simulink model "DSPB_MB_SS"  (Simulink 8.1)
settings: Solver=VariableStepDiscrete  StartTime=0.0  StopTime=DSPB_MB_SS_param.endTime  RelTol=1e-3
PreLoadFcn:
  | % Run the setup script when the model is opened
  | setup_DSPB_MB_SS;
InitFcn:
  | % Run the setup script again just before the
  | % model is run, so that any updates made
  | % after opening are applied.
  | setup_DSPB_MB_SS;
undefined symbols (not defined in the file or in its folder): a, AdvDSPBDMemDisplay, dpoly, DSPB_MB_SS_param, dspba, evalAionMaskParam, primtype, UseDontCare, value, x, y
libraries: DSPBAPrim x298, DspbAdvFftLibrary x34, DSPBABase x5, simulink x3, DSPBAModelBus x3, DSPBAVectorUtil x3, DSPBAControl x2
(part 2 of 4)

== system DSPB_MB_SS/dut/Output_Interface/addr_counter1 ==
  en : Inport
  CmpEQ : DSPBAPrim/CmpEQ  primtype=cmpeq  nInputs=2  nOutputs=1  omode=boolean  otype=sfix(16)  scale=2^-15  rndmethod=Unbiased  factor=1  satmethod=Symmetric  shift_vec=[0 1 2 -1]  value=0  inPortNames=[' '; ' ';]  outPortNames=[' ']  dspbaimage=dspba_prim.jpg  text=fprintf('==');  style=Optimised  visibilities=0  advOptions=[]  version=20130117
  Const1 : DSPBAPrim/Const  primtype=const  nInputs=0  nOutputs=1  omode=Specify via dialog  otype=ufix(DSPB_MB_SS_param.FS+1)  scale=2^-0  rndmethod=Unbiased  factor=1  satmethod=Symmetric  shift_vec=[0 1 2 -1]  value=2^(DSPB_MB_SS_param.FS) + 1  inPortNames=['+'; '+';]  outPortNames=[' ']  dspbaimage=dspba_prim.jpg  text=fprintf('%s', num2str(value));  style=Optimised  visibilities=8 + 1024  floatPrecision=float32_m23  version=20120820
  Const2 : DSPBAPrim/Const  primtype=const  nInputs=0  nOutputs=1  omode=Specify via dialog  otype=ufix(DSPB_MB_SS_param.FS + 1)  scale=2^-0  rndmethod=Unbiased  factor=1  satmethod=Symmetric  shift_vec=[0 1 2 -1]  value=2^(DSPB_MB_SS_param.FS)  inPortNames=['+'; '+';]  outPortNames=[' ']  dspbaimage=dspba_prim.jpg  text=fprintf('%s', num2str(value));  style=Optimised  visibilities=8 + 1024  floatPrecision=float32_m23  version=20120820
  Const3 : DSPBAPrim/Const  primtype=const  nInputs=0  nOutputs=1  omode=boolean  otype=ufix(10)  scale=2^-0  rndmethod=Unbiased  factor=1  satmethod=Symmetric  shift_vec=[0 1 2 -1]  value=1  inPortNames=['+'; '+';]  outPortNames=[' ']  dspbaimage=dspba_prim.jpg  text=fprintf('%s', num2str(value));  style=Optimised  visibilities=8 + 1024  floatPrecision=float32_m23  version=20120820
  Const4 : DSPBAPrim/Const  primtype=const  nInputs=0  nOutputs=1  omode=Inherit via internal rule  otype=ufix(10)  scale=2^-0  rndmethod=Unbiased  factor=1  satmethod=Symmetric  shift_vec=[0 1 2 -1]  value=0  inPortNames=['+'; '+';]  outPortNames=[' ']  dspbaimage=dspba_prim.jpg  text=fprintf('%s', num2str(value));  style=Optimised  visibilities=8 + 1024  floatPrecision=float32_m23  version=20120820
  LoadableCounter : DSPBAPrim/LoadableCounter  primtype=loadablecounter  nInputs=5  nOutputs=1  omode=Specify via dialog  otype=ufix(DSPB_MB_SS_param.FS+1)  scale=2^-0  rndmethod=Unbiased  factor=1  satmethod=Symmetric  shift_vec=[0 1 2 -1]  value=[0 2^(DSPB_MB_SS_param.FS) + 1 1]  inPortNames=['en';'ld';'i ';'s ';'m ']  outPortNames=[' ']  dspbaimage=dspba_prim.jpg  text=fprintf('loadable\ncounter\n[%d %d %d]', value(1), value(2), value(3));  style=Optimised  visibilities=8 + 1024  version=20090407
  SampleDelay : DSPBAPrim/SampleDelay  primtype=sampdelay  nInputs=1  nOutputs=1  omode=Inherit via internal rule  otype=sfix(16)  scale=2^-15  rndmethod=Unbiased  factor=1  satmethod=Symmetric  shift_vec=[0 1 2 -1]  value=1  inPortNames=[' '; ' ';]  outPortNames=[' ']  dspbaimage=dspba_prim.jpg  text=dpoly(1, eye(1,value+1), 'z')  style=Optimised  visibilities=8 + 1024 + 2^17 + 2^18  flexible=off  slackgroup=0  augmented=0  version=20090407  advOptions=[]
  count : Outport
  wires:
  Const2/1 -> CmpEQ/2
  CmpEQ/1 -> SampleDelay/1
  Const4/1 -> LoadableCounter/3
  Const1/1 -> LoadableCounter/5
  SampleDelay/1 -> LoadableCounter/2
  Const3/1 -> LoadableCounter/4
  en/1 -> LoadableCounter/1
  LoadableCounter/1 -> count/1, CmpEQ/1

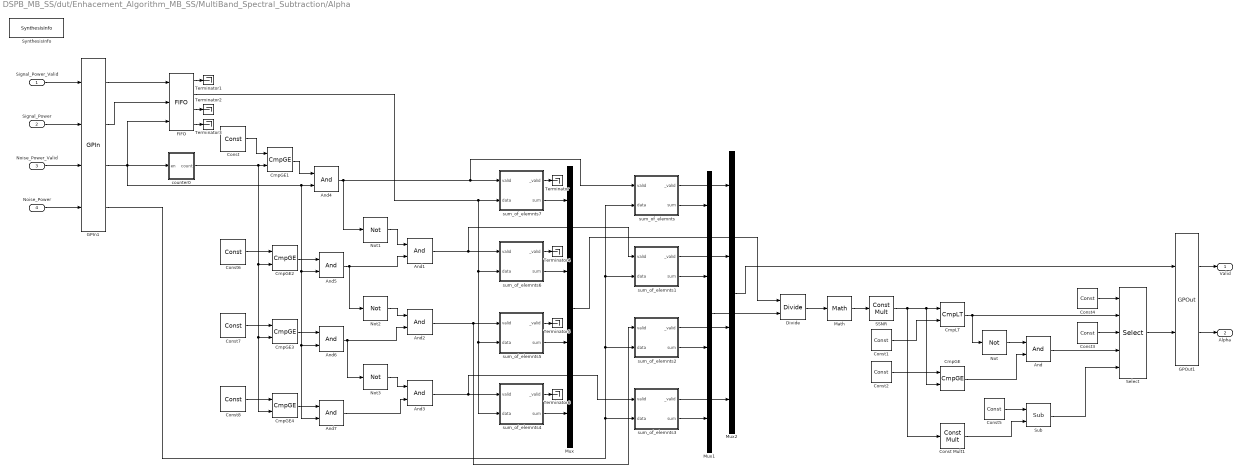
== system DSPB_MB_SS/dut/Enhacement_Algorithm_MB_SS/MultiBand_Spectral_Subtraction/Alpha ==
  Signal_Power_Valid : Inport
  Signal_Power : Inport  Port=2
  Noise_Power_Valid : Inport  Port=3
  Noise_Power : Inport  Port=4
  And{,1..7} (8 alike) : DSPBAPrim/And  primtype=and  nInputs=2  nOutputs=1  omode=Inherit via internal rule  otype=sfix(16)  scale=2^-15  rndmethod=Unbiased  factor=1  satmethod=Symmetric  shift_vec=[0 1 2 -1]  value=0  inPortNames=[' '; ' '; ' '; ' '; ' '; ' '; ' '; ' '; ' '; ' '; ' '; ' '; ' '; ' '; ' '; ' '; ]  outPortNames=[' ']  dspbaimage=dspba_prim.jpg  text=fprintf('&');  style=Optimised  visibilities=8+2  version=20090407
  CmpGE{,1..4} (5 alike) : DSPBAPrim/CmpGE  primtype=cmpgte  nInputs=2  nOutputs=1  omode=boolean  otype=sfix(16)  scale=2^-15  rndmethod=Unbiased  factor=1  satmethod=Symmetric  shift_vec=[0 1 2 -1]  value=0  inPortNames=['a'; 'b';]  outPortNames=[' ']  dspbaimage=dspba_prim.jpg  text=fprintf('a>=b');  style=Optimised  visibilities=0  advOptions=[]  version=20130117
  CmpLT : DSPBAPrim/CmpLT  primtype=cmplt  nInputs=2  nOutputs=1  omode=boolean  otype=sfix(16)  scale=2^-15  rndmethod=Unbiased  factor=1  satmethod=Symmetric  shift_vec=[0 1 2 -1]  value=0  inPortNames=['a'; 'b';]  outPortNames=[' ']  dspbaimage=dspba_prim.jpg  text=fprintf('a<b');  style=Optimised  visibilities=0  advOptions=[]  version=20130117
  Const : DSPBAPrim/Const  primtype=const  nInputs=0  nOutputs=1  omode=Specify via dialog  otype=ufix(10)  scale=2^-0  rndmethod=Unbiased  factor=1  satmethod=Symmetric  shift_vec=[0 1 2 -1]  value=2^(DSPB_MB_SS_param.FS-1-log2(DSPB_MB_SS_param.NB))  inPortNames=['+'; '+';]  outPortNames=[' ']  dspbaimage=dspba_prim.jpg  text=fprintf('%s', num2str(value));  style=Optimised  visibilities=8 + 1024  floatPrecision=float32_m23  version=20120820
  Const Mult1 : DSPBAPrim/Const Mult  primtype=constmult  nInputs=1  nOutputs=1  omode=Inherit via internal rule  otype=sfix(16)  scale=2^-15  rndmethod=Unbiased  factor=1  satmethod=Symmetric  shift_vec=[0 1 2 -1]  value=3/20  inPortNames=[' '; ' ';]  outPortNames=[' ']  dspbaimage=dspba_prim.jpg  text=fprintf('cx');  style=Optimised  visibilities=8+2^10+2^17+2^18  floatRounding=correct  advOptions=[]  version=20140218
  Const1 : DSPBAPrim/Const  primtype=const  nInputs=0  nOutputs=1  omode=single  otype=sfix(16)  scale=2^-15  rndmethod=Unbiased  factor=1  satmethod=Symmetric  shift_vec=[0 1 2 -1]  value=-5  inPortNames=['+'; '+';]  outPortNames=[' ']  dspbaimage=dspba_prim.jpg  text=fprintf('%s', num2str(value));  style=Optimised  visibilities=8 + 1024  floatPrecision=float32_m23  version=20120820
  Const2 : DSPBAPrim/Const  primtype=const  nInputs=0  nOutputs=1  omode=single  otype=sfix(16)  scale=2^-15  rndmethod=Unbiased  factor=1  satmethod=Symmetric  shift_vec=[0 1 2 -1]  value=20  inPortNames=['+'; '+';]  outPortNames=[' ']  dspbaimage=dspba_prim.jpg  text=fprintf('%s', num2str(value));  style=Optimised  visibilities=8 + 1024  floatPrecision=float32_m23  version=20120820
  Const3 : DSPBAPrim/Const  primtype=const  nInputs=0  nOutputs=1  omode=single  otype=sfix(16)  scale=2^-15  rndmethod=Unbiased  factor=1  satmethod=Symmetric  shift_vec=[0 1 2 -1]  value=5  inPortNames=['+'; '+';]  outPortNames=[' ']  dspbaimage=dspba_prim.jpg  text=fprintf('%s', num2str(value));  style=Optimised  visibilities=8 + 1024  floatPrecision=float32_m23  version=20120820
  Const4 : DSPBAPrim/Const  primtype=const  nInputs=0  nOutputs=1  omode=single  otype=sfix(16)  scale=2^-15  rndmethod=Unbiased  factor=1  satmethod=Symmetric  shift_vec=[0 1 2 -1]  value=1  inPortNames=['+'; '+';]  outPortNames=[' ']  dspbaimage=dspba_prim.jpg  text=fprintf('%s', num2str(value));  style=Optimised  visibilities=8 + 1024  floatPrecision=float32_m23  version=20120820
  Const5 : DSPBAPrim/Const  primtype=const  nInputs=0  nOutputs=1  omode=single  otype=sfix(16)  scale=2^-15  rndmethod=Unbiased  factor=1  satmethod=Symmetric  shift_vec=[0 1 2 -1]  value=4  inPortNames=['+'; '+';]  outPortNames=[' ']  dspbaimage=dspba_prim.jpg  text=fprintf('%s', num2str(value));  style=Optimised  visibilities=8 + 1024  floatPrecision=float32_m23  version=20120820
  Const6 : DSPBAPrim/Const  primtype=const  nInputs=0  nOutputs=1  omode=Specify via dialog  otype=ufix(10)  scale=2^-0  rndmethod=Unbiased  factor=1  satmethod=Symmetric  shift_vec=[0 1 2 -1]  value=2*2^(DSPB_MB_SS_param.FS-1-log2(DSPB_MB_SS_param.NB))  inPortNames=['+'; '+';]  outPortNames=[' ']  dspbaimage=dspba_prim.jpg  text=fprintf('%s', num2str(value));  style=Optimised  visibilities=8 + 1024  floatPrecision=float32_m23  version=20120820
  Const7 : DSPBAPrim/Const  primtype=const  nInputs=0  nOutputs=1  omode=Specify via dialog  otype=ufix(10)  scale=2^-0  rndmethod=Unbiased  factor=1  satmethod=Symmetric  shift_vec=[0 1 2 -1]  value=3*2^(DSPB_MB_SS_param.FS-1-log2(DSPB_MB_SS_param.NB))  inPortNames=['+'; '+';]  outPortNames=[' ']  dspbaimage=dspba_prim.jpg  text=fprintf('%s', num2str(value));  style=Optimised  visibilities=8 + 1024  floatPrecision=float32_m23  version=20120820
  Const8 : DSPBAPrim/Const  primtype=const  nInputs=0  nOutputs=1  omode=Specify via dialog  otype=ufix(10)  scale=2^-0  rndmethod=Unbiased  factor=1  satmethod=Symmetric  shift_vec=[0 1 2 -1]  value=4*2^(DSPB_MB_SS_param.FS-1-log2(DSPB_MB_SS_param.NB))  inPortNames=['+'; '+';]  outPortNames=[' ']  dspbaimage=dspba_prim.jpg  text=fprintf('%s', num2str(value));  style=Optimised  visibilities=8 + 1024  floatPrecision=float32_m23  version=20120820
  Divide : DSPBAPrim/Divide  primtype=divide  nInputs=2  nOutputs=1  omode=Inherit via internal rule  otype=sfix(16)  scale=2^-15  rndmethod=Unbiased  factor=1  satmethod=Symmetric  shift_vec=[0 1 2 -1]  value=round([0:255]/17)  inPortNames=[' '; ' ';]  outPortNames=[' ']  dspbaimage=dspba_prim.jpg  text=fprintf('a\n----\nb');  style=Optimised  visibilities=8+2^17+2^18  floatRounding=correct  advOptions=[]  version=20130115
  FIFO : DSPBAPrim/FIFO  primtype=fifo  nInputs=3  nOutputs=4  omode=Inherit via internal rule  otype=sfix(16)  scale=2^-15  rndmethod=Unbiased  factor=1  satmethod=Symmetric  shift_vec=[0 1 2 -1]  value=[2^(DSPB_MB_SS_param.FS-1) 1 2^(DSPB_MB_SS_param.FS-1)]  inPortNames=['w'; 'd'; 'r'; 'f']  outPortNames=['v'; 'q'; 't'; 'f']  dspbaimage=dspba_prim.jpg  text=fprintf('fifo');  style=Optimised  visibilities=263168  version=20130808  user_sclr=off
  GPIn1 : DSPBAPrim/GPIn  primtype=gpin  nInputs=evalAionMaskParam(gcb,'value',1)  nOutputs=evalAionMaskParam(gcb,'value',1)  omode=Inherit via internal rule  otype=sfix(16)  scale=2^-15  rndmethod=Unbiased  factor=1  satmethod=Symmetric  shift_vec=[0 1 2 -1]  value=4  inPortNames=[' ' ' ' ' ' ' ' ' ' ' ' ' ' ' ' ' ' ' ' ' ' ' ' ' ' ' ' ' ' ' ' ' ' ' ' ' ' ' ' ' ' ' ' ' ' ' ' ' ' ' ' ' ' ' ' ' ' ' ' ' ' ' ' ' ' ' ' ' ']'  outPortNames=[' ' ' ' ' ' ' ' ' ' ' ' ' ' ' ' ' ' ' ' ' ' ' ' ' ' ' ' ' ' ' ' ' ' ' ' ' ' ' ' ' ' ' ' ' ' ' ' ' ' ' ' ' ' ' ' ' ' ' ' ' ' ' ' ' ' ' ' ' ']'  dspbaimage=dspba_prim.jpg  text=fprintf('GPIn');  style=Optimised  visibilities=1024  latencyCorrection=0  scheduleOrigin=on  version=20090407
  GPOut1 : DSPBAPrim/GPOut  primtype=gpout  nInputs=evalAionMaskParam(gcb,'value',1)  nOutputs=evalAionMaskParam(gcb,'value',1)  omode=Inherit via internal rule  otype=sfix(16)  scale=2^-15  rndmethod=Unbiased  factor=1  satmethod=Symmetric  shift_vec=[0 1 2 -1]  value=2  inPortNames=[' ' ' ' ' ' ' ' ' ' ' ' ' ' ' ' ' ' ' ' ' ' ' ' ' ' ' ' ' ' ' ' ' ' ' ' ' ' ' ' ' ' ' ' ' ' ' ' ' ' ' ' ' ' ' ' ' ' ' ' ' ' ' ' ' ' ' ' ' ']'  outPortNames=[' ' ' ' ' ' ' ' ' ' ' ' ' ' ' ' ' ' ' ' ' ' ' ' ' ' ' ' ' ' ' ' ' ' ' ' ' ' ' ' ' ' ' ' ' ' ' ' ' ' ' ' ' ' ' ' ' ' ' ' ' ' ' ' ' ' ' ' ' ']'  dspbaimage=dspba_prim.jpg  text=fprintf('GPOut');  style=Optimised  visibilities=1024  latencyCorrection=0  version=20090407
  Math : DSPBAPrim/Math  primtype=mathfunc  nInputs=1  nOutputs=1  omode=Inherit via internal rule  otype=sfix(16)  scale=2^-15  rndmethod=Unbiased  factor=1  satmethod=Symmetric  shift_vec=[0 1 2 -1]  value=round([0:255]/17)  inPortNames=[' '; ' ';]  outPortNames=[' ']  dspbaimage=dspba_prim_float.jpg  text=fprintf('exp(x)');  style=Optimised  visibilities=2^17  functionExpr=log10(x)  advOptions=[]  floatRounding=correct  version=20130910
  Mux : Mux
  Mux1 : Mux
  Mux2 : Mux
  Not{,1..3} (4 alike) : DSPBAPrim/Not  primtype=not  nInputs=1  nOutputs=1  omode=Inherit via internal rule  otype=sfix(16)  scale=2^-15  rndmethod=Unbiased  factor=1  satmethod=Symmetric  shift_vec=[0 1 2 -1]  value=0  inPortNames=[' '; ' ';]  outPortNames=[' ']  dspbaimage=dspba_prim.jpg  text=fprintf('~');  style=Optimised  visibilities=8  version=20090407
  SSNR : DSPBAPrim/Const Mult  primtype=constmult  nInputs=1  nOutputs=1  omode=Inherit via internal rule  otype=sfix(16)  scale=2^-15  rndmethod=Unbiased  factor=1  satmethod=Symmetric  shift_vec=[0 1 2 -1]  value=10  inPortNames=[' '; ' ';]  outPortNames=[' ']  dspbaimage=dspba_prim.jpg  text=fprintf('cx');  style=Optimised  visibilities=8+2^10+2^17+2^18  floatRounding=correct  advOptions=[]  version=20140218
  Select : DSPBAPrim/Select  primtype=select  nInputs=str2num(get_param(gcb,'value'))*2+1  nOutputs=1  omode=Inherit via internal rule  otype=sfix(16)  scale=2^-15  rndmethod=Unbiased  factor=1  satmethod=Symmetric  shift_vec=[0 1 2 -1]  value=2  inPortNames=['d'; '0'; 'a'; '1'; 'b'; '2'; 'c'; '3'; 'd'; '4'; 'e'; '5'; 'f'; '6'; 'g'; '7'; 'h'; '8'; 'i'; '9'; 'j']  outPortNames=[' ']  dspbaimage=dspba_prim.jpg  text=fprintf('%s', primtype);  style=Optimised  visibilities=8 + 1024  version=20090407
  Sub : DSPBAPrim/Sub  primtype=sub  nInputs=2  nOutputs=1  omode=Inherit via internal rule with word growth  otype=sfix(16)  scale=2^-15  rndmethod=Unbiased  factor=1  satmethod=Symmetric  shift_vec=[0 1 2 -1]  value=0  inPortNames=['+'; '-';]  outPortNames=[' ']  dspbaimage=dspba_prim.jpg  text=fprintf('-');  style=Optimised  visibilities=8+2^17+2^18  floatRounding=correct  advOptions=[]  version=20130115
  SynthesisInfo : DSPBAPrim/SynthesisInfo  primtype=synthinfo  nInputs=0  nOutputs=0  omode=Inherit via internal rule  otype=sfix(16)  scale=2^-15  rndmethod=Truncate  factor=1  satmethod=Symmetric  shift_vec=[0 1 2 -1]  value=99  inPortNames=[' '; ' ';]  outPortNames=[' ']  dspbaimage=dspba_prim_ctrl.jpg  text=fprintf('Style=%s', style);  style=Scheduled  visibilities=2^17+2^18+2^19+2^20  constraintInUse=off  constraintRelation==  constraintLimit=5  bitAccurate=on  version=20150220
  Terminator{,1..6} (7 alike) : Terminator
  counter0 : Subsystem
  sum_of_elemnts : Subsystem
  sum_of_elemnts1 : Subsystem
  sum_of_elemnts2 : Subsystem
  sum_of_elemnts3 : Subsystem
  sum_of_elemnts4 : Subsystem
  sum_of_elemnts5 : Subsystem
  sum_of_elemnts6 : Subsystem
  sum_of_elemnts7 : Subsystem
  Valid : Outport
  Alpha : Outport  Port=2
  wires:
  Math/1 -> SSNR/1
  SSNR/1 -> Const Mult1/1, CmpGE/2, CmpLT/1
  Const1/1 -> CmpLT/2
  CmpLT/1 -> Not/1, Select/2
  Const2/1 -> CmpGE/1
  Not/1 -> And/1
  CmpGE/1 -> And/2
  And/1 -> Select/4
  Const3/1 -> Select/3
  Const4/1 -> Select/1
  Const5/1 -> Sub/1
  Const Mult1/1 -> Sub/2
  Sub/1 -> Select/5
  Signal_Power_Valid/1 -> GPIn1/1
  Signal_Power/1 -> GPIn1/2
  Noise_Power/1 -> GPIn1/4
  Noise_Power_Valid/1 -> GPIn1/3
  GPIn1/2 -> FIFO/2
  GPIn1/1 -> FIFO/1
  Const/1 -> CmpGE1/1
  counter0/1(count) -> CmpGE1/2, CmpGE2/2, CmpGE4/2, CmpGE3/2
  GPIn1/3 -> And7/2, And6/2, And5/2, And4/2, counter0/1(en), FIFO/3
  Not1/1 -> And1/1
  Not2/1 -> And2/1
  Const6/1 -> CmpGE2/1
  Const7/1 -> CmpGE3/1
  And5/1 -> And1/2, Not2/1
  Not3/1 -> And3/1
  CmpGE2/1 -> And5/1
  And6/1 -> Not3/1, And2/2
  And7/1 -> And3/2
  CmpGE3/1 -> And6/1
  CmpGE4/1 -> And7/1
  Const8/1 -> CmpGE4/1
  CmpGE1/1 -> And4/1
  And4/1 -> Not1/1, sum_of_elemnts7/1(valid), sum_of_elemnts/1(valid)
  And1/1 -> sum_of_elemnts6/1(valid), sum_of_elemnts1/1(valid)
  And2/1 -> sum_of_elemnts5/1(valid), sum_of_elemnts2/1(valid)
  And3/1 -> sum_of_elemnts4/1(valid), sum_of_elemnts3/1(valid)
  FIFO/2 -> sum_of_elemnts7/2(data), sum_of_elemnts6/2(data), sum_of_elemnts5/2(data), sum_of_elemnts4/2(data)
  GPIn1/4 -> sum_of_elemnts3/2(data), sum_of_elemnts2/2(data), sum_of_elemnts1/2(data), sum_of_elemnts/2(data)
  Divide/1 -> Math/1
  FIFO/1 -> Terminator1/1
  FIFO/3 -> Terminator2/1
  FIFO/4 -> Terminator3/1
  sum_of_elemnts7/2(sum) -> Mux/1
  sum_of_elemnts6/2(sum) -> Mux/2
  sum_of_elemnts4/2(sum) -> Mux/4
  sum_of_elemnts5/2(sum) -> Mux/3
  sum_of_elemnts/2(sum) -> Mux1/1
  sum_of_elemnts3/2(sum) -> Mux1/4
  sum_of_elemnts2/2(sum) -> Mux1/3
  sum_of_elemnts1/2(sum) -> Mux1/2
  Mux/1 -> Divide/1
  Mux1/1 -> Divide/2
  sum_of_elemnts7/1(_valid) -> Terminator/1
  sum_of_elemnts6/1(_valid) -> Terminator4/1
  sum_of_elemnts5/1(_valid) -> Terminator5/1
  sum_of_elemnts4/1(_valid) -> Terminator6/1
  GPOut1/1 -> Valid/1
  GPOut1/2 -> Alpha/1
  Select/1 -> GPOut1/2
  sum_of_elemnts/1(_valid) -> Mux2/1
  sum_of_elemnts1/1(_valid) -> Mux2/2
  sum_of_elemnts2/1(_valid) -> Mux2/3
  sum_of_elemnts3/1(_valid) -> Mux2/4
  Mux2/1 -> GPOut1/1

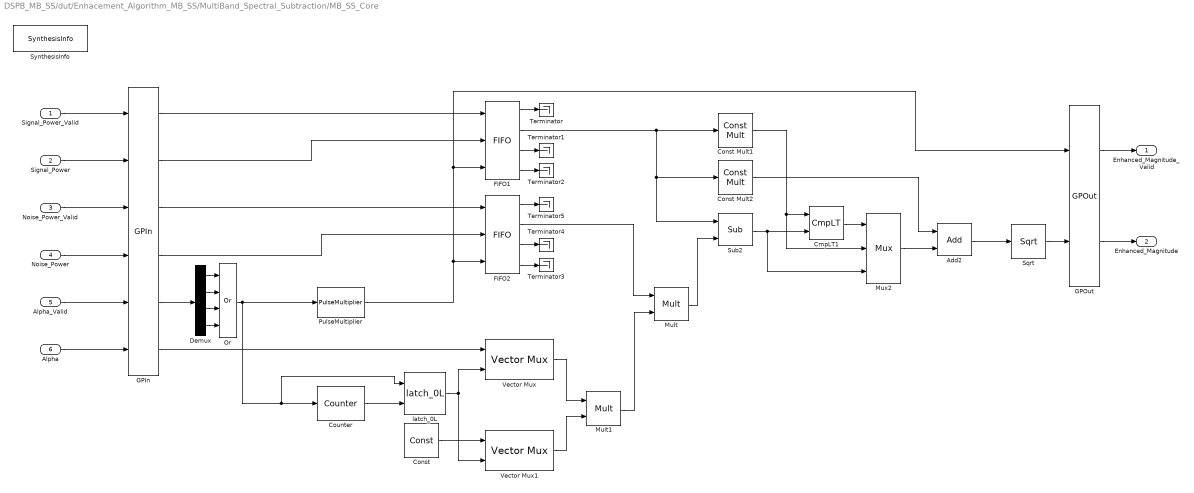
== system DSPB_MB_SS/dut/Enhacement_Algorithm_MB_SS/MultiBand_Spectral_Subtraction/MB_SS_Core ==
  Signal_Power_Valid : Inport
  Signal_Power : Inport  Port=2
  Noise_Power_Valid : Inport  Port=3
  Noise_Power : Inport  Port=4
  Alpha_Valid : Inport  Port=5
  Alpha : Inport  Port=6
  Add2 : DSPBAPrim/Add  primtype=add  nInputs=evalAionMaskParam(gcb,'value',1)  nOutputs=1  omode=Inherit via internal rule  otype=ufix(DSPB_MB_SS_param.FS + 1)  scale=2^-0  rndmethod=Unbiased  factor=1  satmethod=Symmetric  shift_vec=[0 1 2 -1]  value=2  inPortNames=[' '; ' ';]  outPortNames=[' ']  dspbaimage=dspba_prim.jpg  text=fprintf('+');  style=Optimised  visibilities=1032+2^17+2^18+2^19  genFPC=off  floatRounding=correct  advOptions=[]  version=20130821
  CmpLT1 : DSPBAPrim/CmpLT  primtype=cmplt  nInputs=2  nOutputs=1  omode=boolean  otype=sfix(16)  scale=2^-15  rndmethod=Unbiased  factor=1  satmethod=Symmetric  shift_vec=[0 1 2 -1]  value=0  inPortNames=['a'; 'b';]  outPortNames=[' ']  dspbaimage=dspba_prim.jpg  text=fprintf('a<b');  style=Optimised  visibilities=0  advOptions=[]  version=20130117
  Const : DSPBAPrim/Const  primtype=const  nInputs=0  nOutputs=1  omode=single  otype=sfix(16)  scale=2^-15  rndmethod=Unbiased  factor=1  satmethod=Symmetric  shift_vec=[0 1 2 -1]  value=[1 2.5 2.5 1.5]  inPortNames=['+'; '+';]  outPortNames=[' ']  dspbaimage=dspba_prim.jpg  text=fprintf('%s', num2str(value));  style=Optimised  visibilities=8 + 1024  floatPrecision=float32_m23  version=20120820
  Const Mult1 : DSPBAPrim/Const Mult  primtype=constmult  nInputs=1  nOutputs=1  omode=Inherit via internal rule  otype=sfix(16)  scale=2^-15  rndmethod=Unbiased  factor=1  satmethod=Symmetric  shift_vec=[0 1 2 -1]  value=0.002  inPortNames=[' '; ' ';]  outPortNames=[' ']  dspbaimage=dspba_prim.jpg  text=fprintf('cx');  style=Optimised  visibilities=8+2^10+2^17+2^18  floatRounding=correct  advOptions=[]  version=20140218
  Const Mult2 : DSPBAPrim/Const Mult  primtype=constmult  nInputs=1  nOutputs=1  omode=Inherit via internal rule  otype=sfix(16)  scale=2^-15  rndmethod=Unbiased  factor=1  satmethod=Symmetric  shift_vec=[0 1 2 -1]  value=0.05  inPortNames=[' '; ' ';]  outPortNames=[' ']  dspbaimage=dspba_prim.jpg  text=fprintf('cx');  style=Optimised  visibilities=8+2^10+2^17+2^18  floatRounding=correct  advOptions=[]  version=20140218
  Counter : DSPBAPrim/Counter  primtype=counter  nInputs=1  nOutputs=1  omode=Inherit via internal rule  otype=ufix(16)  scale=2^-0  rndmethod=Unbiased  factor=1  satmethod=Symmetric  shift_vec=[0 1 2 -1]  value=[DSPB_MB_SS_param.NB-1 DSPB_MB_SS_param.NB 1]  inPortNames=[' '; ' ';]  outPortNames=[' ']  dspbaimage=dspba_prim.jpg  text=fprintf('counter\n[%d %d %d]', value(1), value(2), value(3));  style=Optimised  visibilities=8 + 1024  version=20090407
  Demux : Demux
  FIFO1 : DSPBAPrim/FIFO  primtype=fifo  nInputs=3  nOutputs=4  omode=Inherit via internal rule  otype=sfix(16)  scale=2^-15  rndmethod=Unbiased  factor=1  satmethod=Symmetric  shift_vec=[0 1 2 -1]  value=[2^(DSPB_MB_SS_param.FS-1) 1 2^(DSPB_MB_SS_param.FS-1)]  inPortNames=['w'; 'd'; 'r'; 'f']  outPortNames=['v'; 'q'; 't'; 'f']  dspbaimage=dspba_prim.jpg  text=fprintf('fifo');  style=Optimised  visibilities=263168  version=20130808  user_sclr=off
  FIFO2 : DSPBAPrim/FIFO  primtype=fifo  nInputs=3  nOutputs=4  omode=Inherit via internal rule  otype=sfix(16)  scale=2^-15  rndmethod=Unbiased  factor=1  satmethod=Symmetric  shift_vec=[0 1 2 -1]  value=[2^(DSPB_MB_SS_param.FS-1) 1 2^(DSPB_MB_SS_param.FS-1)]  inPortNames=['w'; 'd'; 'r'; 'f']  outPortNames=['v'; 'q'; 't'; 'f']  dspbaimage=dspba_prim.jpg  text=fprintf('fifo');  style=Optimised  visibilities=263168  version=20130808  user_sclr=off
  GPIn : DSPBAPrim/GPIn  primtype=gpin  nInputs=evalAionMaskParam(gcb,'value',1)  nOutputs=evalAionMaskParam(gcb,'value',1)  omode=Inherit via internal rule  otype=sfix(16)  scale=2^-15  rndmethod=Unbiased  factor=1  satmethod=Symmetric  shift_vec=[0 1 2 -1]  value=6  inPortNames=[' ' ' ' ' ' ' ' ' ' ' ' ' ' ' ' ' ' ' ' ' ' ' ' ' ' ' ' ' ' ' ' ' ' ' ' ' ' ' ' ' ' ' ' ' ' ' ' ' ' ' ' ' ' ' ' ' ' ' ' ' ' ' ' ' ' ' ' ' ']'  outPortNames=[' ' ' ' ' ' ' ' ' ' ' ' ' ' ' ' ' ' ' ' ' ' ' ' ' ' ' ' ' ' ' ' ' ' ' ' ' ' ' ' ' ' ' ' ' ' ' ' ' ' ' ' ' ' ' ' ' ' ' ' ' ' ' ' ' ' ' ' ' ']'  dspbaimage=dspba_prim.jpg  text=fprintf('GPIn');  style=Optimised  visibilities=1024  latencyCorrection=0  scheduleOrigin=on  version=20090407
  GPOut : DSPBAPrim/GPOut  primtype=gpout  nInputs=evalAionMaskParam(gcb,'value',1)  nOutputs=evalAionMaskParam(gcb,'value',1)  omode=Inherit via internal rule  otype=sfix(16)  scale=2^-15  rndmethod=Unbiased  factor=1  satmethod=Symmetric  shift_vec=[0 1 2 -1]  value=2  inPortNames=[' ' ' ' ' ' ' ' ' ' ' ' ' ' ' ' ' ' ' ' ' ' ' ' ' ' ' ' ' ' ' ' ' ' ' ' ' ' ' ' ' ' ' ' ' ' ' ' ' ' ' ' ' ' ' ' ' ' ' ' ' ' ' ' ' ' ' ' ' ']'  outPortNames=[' ' ' ' ' ' ' ' ' ' ' ' ' ' ' ' ' ' ' ' ' ' ' ' ' ' ' ' ' ' ' ' ' ' ' ' ' ' ' ' ' ' ' ' ' ' ' ' ' ' ' ' ' ' ' ' ' ' ' ' ' ' ' ' ' ' ' ' ' ']'  dspbaimage=dspba_prim.jpg  text=fprintf('GPOut');  style=Optimised  visibilities=1024  latencyCorrection=0  version=20090407
  Mult : DSPBAPrim/Mult  primtype=mult  nInputs=2  nOutputs=1  omode=Inherit via internal rule  otype=sfix(16)  scale=2^-15  rndmethod=Unbiased  factor=1  satmethod=Symmetric  shift_vec=[0 1 2 -1]  value=0  inPortNames=[' '; ' ';]  outPortNames=[' ']  dspbaimage=dspba_prim.jpg  text=fprintf('X');  style=Optimised  visibilities=8+2^18+2^19  floatPrecision=float32_m23  floatRounding=correct  advOptions=[]  version=20130115
  Mult1 : DSPBAPrim/Mult  primtype=mult  nInputs=2  nOutputs=1  omode=Inherit via internal rule  otype=sfix(16)  scale=2^-15  rndmethod=Unbiased  factor=1  satmethod=Symmetric  shift_vec=[0 1 2 -1]  value=0  inPortNames=[' '; ' ';]  outPortNames=[' ']  dspbaimage=dspba_prim.jpg  text=fprintf('X');  style=Optimised  visibilities=8+2^18+2^19  floatPrecision=float32_m23  floatRounding=correct  advOptions=[]  version=20130115
  Mux2 : DSPBAPrim/Mux  primtype=mux  nInputs=evalAionMaskParam(gcb,'value',1)+1  nOutputs=1  omode=Inherit via internal rule  otype=sfix(16)  scale=2^-15  rndmethod=Unbiased  factor=1  satmethod=Symmetric  shift_vec=[0 1 2 -1]  value=2  inPortNames=['s '; 'd0'; 'd1'; 'd2'; 'd3'; 'd4'; 'd5'; 'd6'; 'd7'; 'd8'; 'd9';]  outPortNames=[' ']  dspbaimage=dspba_prim.jpg  text=fprintf('%s', primtype);  style=Optimised  visibilities=1032  version=20131025
  Or : DSPBAPrim/Or  primtype=or  nInputs=4  nOutputs=1  omode=Inherit via internal rule  otype=sfix(16)  scale=2^-15  rndmethod=Unbiased  factor=1  satmethod=Symmetric  shift_vec=[0 1 2 -1]  value=0  inPortNames=[' '; ' '; ' '; ' '; ' '; ' '; ' '; ' '; ' '; ' '; ' '; ' '; ' '; ' '; ' '; ' '; ]  outPortNames=[' ']  dspbaimage=dspba_prim.jpg  text=fprintf('|');  style=Optimised  visibilities=8+2  version=20090407
  PulseMultiplier : DspbAdvFftLibrary/Common/PulseMultiplier  N=DSPB_MB_SS_param.FS-1-log2(DSPB_MB_SS_param.NB)
  Sqrt : DSPBAPrim/Sqrt  primtype=sqrtfunc  nInputs=1  nOutputs=1  omode=Inherit via internal rule  otype=sfix(16)  scale=2^-15  rndmethod=Unbiased  factor=1  satmethod=Symmetric  shift_vec=[0 1 2 -1]  value=round([0:255]/17)  inPortNames=[' '; ' ';]  outPortNames=[' ']  dspbaimage=dspba_prim_float.jpg  text=fprintf('sqrt(x)');  style=Optimised  visibilities=2^17  functionExpr=sqrt(x)  floatRounding=correct  advOptions=[]  version=20120730
  Sub2 : DSPBAPrim/Sub  primtype=sub  nInputs=2  nOutputs=1  omode=Inherit via internal rule with word growth  otype=sfix(16)  scale=2^-15  rndmethod=Unbiased  factor=1  satmethod=Symmetric  shift_vec=[0 1 2 -1]  value=0  inPortNames=['+'; '-';]  outPortNames=[' ']  dspbaimage=dspba_prim.jpg  text=fprintf('-');  style=Optimised  visibilities=8+2^17+2^18  floatRounding=correct  advOptions=[]  version=20130115
  SynthesisInfo : DSPBAPrim/SynthesisInfo  primtype=synthinfo  nInputs=0  nOutputs=0  omode=Inherit via internal rule  otype=sfix(16)  scale=2^-15  rndmethod=Truncate  factor=1  satmethod=Symmetric  shift_vec=[0 1 2 -1]  value=99  inPortNames=[' '; ' ';]  outPortNames=[' ']  dspbaimage=dspba_prim_ctrl.jpg  text=fprintf('Style=%s', style);  style=Scheduled  visibilities=2^17+2^18+2^19+2^20  constraintInUse=off  constraintRelation==  constraintLimit=5  bitAccurate=on  version=20150220
  Terminator{,1..5} (6 alike) : Terminator
  Vector Mux : DSPBAVectorUtil/Vector Mux  vecWidth=DSPB_MB_SS_param.NB
  Vector Mux1 : DSPBAVectorUtil/Vector Mux  vecWidth=DSPB_MB_SS_param.NB
  latch_0L : DSPBAControl/latch_0L
  Enhanced_Magnitude_Valid : Outport
  Enhanced_Magnitude : Outport  Port=2
  wires:
  GPOut/2 -> Enhanced_Magnitude/1
  Signal_Power_Valid/1 -> GPIn/1
  Signal_Power/1 -> GPIn/2
  Noise_Power_Valid/1 -> GPIn/3
  Noise_Power/1 -> GPIn/4
  GPOut/1 -> Enhanced_Magnitude_Valid/1
  Const Mult1/1 -> CmpLT1/1, Mux2/2
  CmpLT1/1 -> Mux2/1
  Mult/1 -> Sub2/2
  Sub2/1 -> CmpLT1/2, Mux2/3
  Mux2/1 -> Add2/2
  Add2/1 -> Sqrt/1
  Const Mult2/1 -> Add2/1
  GPIn/1 -> FIFO1/1
  GPIn/2 -> FIFO1/2
  Alpha/1 -> GPIn/6
  GPIn/3 -> FIFO2/1
  GPIn/4 -> FIFO2/2
  FIFO2/1 -> Terminator5/1
  FIFO2/3 -> Terminator4/1
  FIFO2/4 -> Terminator3/1
  FIFO1/4 -> Terminator2/1
  FIFO1/3 -> Terminator1/1
  FIFO1/1 -> Terminator/1
  Alpha_Valid/1 -> GPIn/5
  GPIn/5 -> Demux/1
  PulseMultiplier/1 -> GPOut/1, FIFO1/3, FIFO2/3
  GPIn/6 -> Vector Mux/1
  latch_0L/1 -> Vector Mux/2, Vector Mux1/2
  Counter/1 -> latch_0L/2
  FIFO2/2 -> Mult/1
  FIFO1/2 -> Sub2/1, Const Mult2/1, Const Mult1/1
  Sqrt/1 -> GPOut/2
  Const/1 -> Vector Mux1/1
  Vector Mux1/1 -> Mult1/2
  Vector Mux/1 -> Mult1/1
  Mult1/1 -> Mult/2
  Demux/3 -> Or/3
  Demux/4 -> Or/4
  Demux/1 -> Or/1
  Demux/2 -> Or/2
  Or/1 -> Counter/1, latch_0L/1, PulseMultiplier/1

== system DSPB_MB_SS/dut/Enhacement_Algorithm_MB_SS/Time_Domain_Reconstruction/IFFT ==
  Input_Valid : Inport
  Input : Inport  Port=2
  Complex to Real-Imag1 : ComplexToRealImag
  Convert : DSPBAPrim/Convert  primtype=convert  nInputs=1  nOutputs=1  omode=single  otype=sfix(16)  scale=2^-15  rndmethod=Biased  factor=1  satmethod=None  shift_vec=[0 1 2 -1]  value=round([0:255]/17)  inPortNames=[' '; ' ';]  outPortNames=[' '; 'c']  dspbaimage=dspba_prim.jpg  text=fprintf('convert');  style=Optimised  visibilities=8+64+256+2^17  clipdetect=off  floatPrecision=float32_m23  advOptions=[]  version=20130211
  FP FFT Light : DspbAdvFftLibrary/Common/FFT_Light  IFFT=true  subchannels=1  br_in=false  N=DSPB_MB_SS_param.FS  in_type=dspba.namedVPFloat('single')  type_strings=dspba.fft.all_float(DSPB_MB_SS_param.FS,dspba.namedVPFloat('single'))  faithful=false  wirecount=1
  GPIn : DSPBAPrim/GPIn  primtype=gpin  nInputs=evalAionMaskParam(gcb,'value',1)  nOutputs=evalAionMaskParam(gcb,'value',1)  omode=Inherit via internal rule  otype=sfix(16)  scale=2^-15  rndmethod=Unbiased  factor=1  satmethod=Symmetric  shift_vec=[0 1 2 -1]  value=2  inPortNames=[' ' ' ' ' ' ' ' ' ' ' ' ' ' ' ' ' ' ' ' ' ' ' ' ' ' ' ' ' ' ' ' ' ' ' ' ' ' ' ' ' ' ' ' ' ' ' ' ' ' ' ' ' ' ' ' ' ' ' ' ' ' ' ' ' ' ' ' ' ']'  outPortNames=[' ' ' ' ' ' ' ' ' ' ' ' ' ' ' ' ' ' ' ' ' ' ' ' ' ' ' ' ' ' ' ' ' ' ' ' ' ' ' ' ' ' ' ' ' ' ' ' ' ' ' ' ' ' ' ' ' ' ' ' ' ' ' ' ' ' ' ' ' ']'  dspbaimage=dspba_prim.jpg  text=fprintf('GPIn');  style=Optimised  visibilities=1024  latencyCorrection=0  scheduleOrigin=on  version=20090407
  GPOut : DSPBAPrim/GPOut  primtype=gpout  nInputs=evalAionMaskParam(gcb,'value',1)  nOutputs=evalAionMaskParam(gcb,'value',1)  omode=Inherit via internal rule  otype=sfix(16)  scale=2^-15  rndmethod=Unbiased  factor=1  satmethod=Symmetric  shift_vec=[0 1 2 -1]  value=2  inPortNames=[' ' ' ' ' ' ' ' ' ' ' ' ' ' ' ' ' ' ' ' ' ' ' ' ' ' ' ' ' ' ' ' ' ' ' ' ' ' ' ' ' ' ' ' ' ' ' ' ' ' ' ' ' ' ' ' ' ' ' ' ' ' ' ' ' ' ' ' ' ']'  outPortNames=[' ' ' ' ' ' ' ' ' ' ' ' ' ' ' ' ' ' ' ' ' ' ' ' ' ' ' ' ' ' ' ' ' ' ' ' ' ' ' ' ' ' ' ' ' ' ' ' ' ' ' ' ' ' ' ' ' ' ' ' ' ' ' ' ' ' ' ' ' ']'  dspbaimage=dspba_prim.jpg  text=fprintf('GPOut');  style=Optimised  visibilities=1024  latencyCorrection=0  version=20090407
  SynthesisInfo : DSPBAPrim/SynthesisInfo  primtype=synthinfo  nInputs=0  nOutputs=0  omode=Inherit via internal rule  otype=sfix(16)  scale=2^-15  rndmethod=Truncate  factor=1  satmethod=Symmetric  shift_vec=[0 1 2 -1]  value=99  inPortNames=[' '; ' ';]  outPortNames=[' ']  dspbaimage=dspba_prim_ctrl.jpg  text=fprintf('Style=%s', style);  style=Scheduled  visibilities=32768  constraintInUse=off  constraintRelation=>  constraintLimit=2  bitAccurate=on  version=20150220
  Terminator : Terminator
  Terminator1 : Terminator
  Terminator2 : Terminator
  Transpose : DspbAdvFftLibrary/Common/Transpose  perm=[fliplr(0:DSPB_MB_SS_param.FS-1)]
  Time_Domain_Output_Valid : Outport
  Time_Domain_Output : Outport  Port=2
  wires:
  Transpose/3 -> Terminator/1
  FP FFT Light/3 -> Terminator1/1
  Input_Valid/1 -> GPIn/1
  Input/1 -> GPIn/2
  GPOut/1 -> Time_Domain_Output_Valid/1
  GPOut/2 -> Time_Domain_Output/1
  GPIn/1 -> FP FFT Light/1
  GPIn/2 -> FP FFT Light/2
  FP FFT Light/1 -> Transpose/1
  FP FFT Light/2 -> Transpose/2
  Transpose/2 -> Convert/1
  Convert/1 -> Complex to Real-Imag1/1
  Complex to Real-Imag1/2 -> Terminator2/1
  Complex to Real-Imag1/1 -> GPOut/2
  Transpose/1 -> GPOut/1

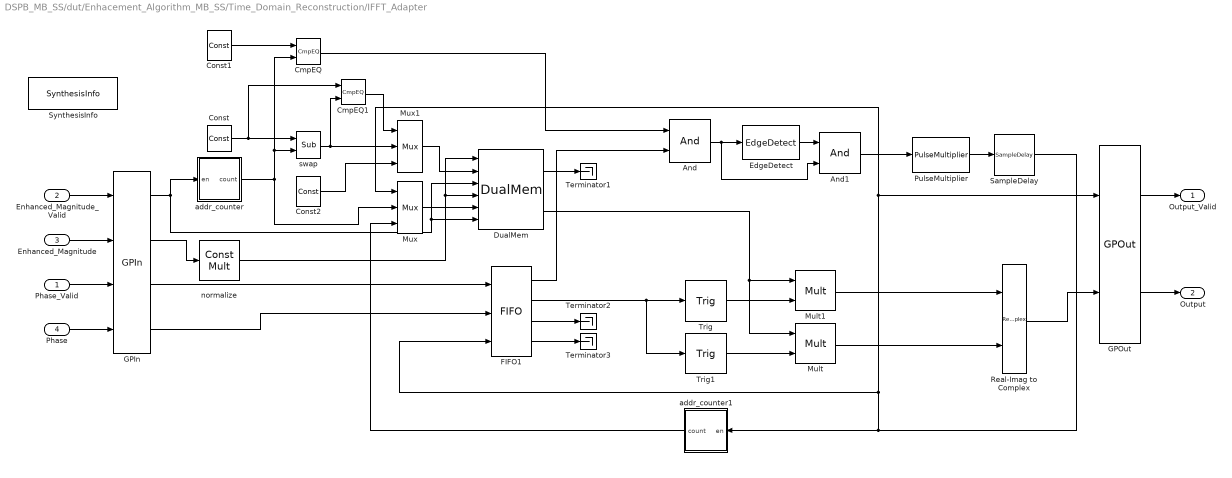
== system DSPB_MB_SS/dut/Enhacement_Algorithm_MB_SS/Time_Domain_Reconstruction/IFFT_Adapter ==
  Phase_Valid : Inport
  Enhanced_Magnitude_Valid : Inport  Port=2
  Enhanced_Magnitude : Inport  Port=3
  Phase : Inport  Port=4
  And : DSPBAPrim/And  primtype=and  nInputs=2  nOutputs=1  omode=Inherit via internal rule  otype=sfix(16)  scale=2^-15  rndmethod=Unbiased  factor=1  satmethod=Symmetric  shift_vec=[0 1 2 -1]  value=0  inPortNames=[' '; ' '; ' '; ' '; ' '; ' '; ' '; ' '; ' '; ' '; ' '; ' '; ' '; ' '; ' '; ' '; ]  outPortNames=[' ']  dspbaimage=dspba_prim.jpg  text=fprintf('&');  style=Optimised  visibilities=8+2  version=20090407
  And1 : DSPBAPrim/And  primtype=and  nInputs=2  nOutputs=1  omode=Inherit via internal rule  otype=sfix(16)  scale=2^-15  rndmethod=Unbiased  factor=1  satmethod=Symmetric  shift_vec=[0 1 2 -1]  value=0  inPortNames=[' '; ' '; ' '; ' '; ' '; ' '; ' '; ' '; ' '; ' '; ' '; ' '; ' '; ' '; ' '; ' '; ]  outPortNames=[' ']  dspbaimage=dspba_prim.jpg  text=fprintf('&');  style=Optimised  visibilities=8+2  version=20090407
  CmpEQ : DSPBAPrim/CmpEQ  primtype=cmpeq  nInputs=2  nOutputs=1  omode=boolean  otype=sfix(16)  scale=2^-15  rndmethod=Unbiased  factor=1  satmethod=Symmetric  shift_vec=[0 1 2 -1]  value=0  inPortNames=[' '; ' ';]  outPortNames=[' ']  dspbaimage=dspba_prim.jpg  text=fprintf('==');  style=Optimised  visibilities=0  advOptions=[]  version=20130117
  CmpEQ1 : DSPBAPrim/CmpEQ  primtype=cmpeq  nInputs=2  nOutputs=1  omode=boolean  otype=sfix(16)  scale=2^-15  rndmethod=Unbiased  factor=1  satmethod=Symmetric  shift_vec=[0 1 2 -1]  value=0  inPortNames=[' '; ' ';]  outPortNames=[' ']  dspbaimage=dspba_prim.jpg  text=fprintf('==');  style=Optimised  visibilities=0  advOptions=[]  version=20130117
  Const : DSPBAPrim/Const  primtype=const  nInputs=0  nOutputs=1  omode=Inherit via internal rule  otype=ufix(DSPB_MB_SS_param.FS+1)  scale=2^-0  rndmethod=Unbiased  factor=1  satmethod=Symmetric  shift_vec=[0 1 2 -1]  value=2^(DSPB_MB_SS_param.FS)  inPortNames=['+'; '+';]  outPortNames=[' ']  dspbaimage=dspba_prim.jpg  text=fprintf('%s', num2str(value));  style=Optimised  visibilities=8 + 1024  floatPrecision=float32_m23  version=20120820
  Const1 : DSPBAPrim/Const  primtype=const  nInputs=0  nOutputs=1  omode=Specify via dialog  otype=ufix(DSPB_MB_SS_param.FS+1)  scale=2^-0  rndmethod=Unbiased  factor=1  satmethod=Symmetric  shift_vec=[0 1 2 -1]  value=2^(DSPB_MB_SS_param.FS-1)-1  inPortNames=['+'; '+';]  outPortNames=[' ']  dspbaimage=dspba_prim.jpg  text=fprintf('%s', num2str(value));  style=Optimised  visibilities=8 + 1024  floatPrecision=float32_m23  version=20120820
  Const2 : DSPBAPrim/Const  primtype=const  nInputs=0  nOutputs=1  omode=Specify via dialog  otype=ufix(DSPB_MB_SS_param.FS+1)  scale=2^-0  rndmethod=Unbiased  factor=1  satmethod=Symmetric  shift_vec=[0 1 2 -1]  value=2^(DSPB_MB_SS_param.FS-1)  inPortNames=['+'; '+';]  outPortNames=[' ']  dspbaimage=dspba_prim.jpg  text=fprintf('%s', num2str(value));  style=Optimised  visibilities=8 + 1024  floatPrecision=float32_m23  version=20120820
  DualMem : DSPBAPrim/DualMem  primtype=dualmem  nInputs=6  nOutputs=2  omode=single  otype=sfix(16)  scale=2^-15  rndmethod=Unbiased  factor=1  satmethod=Symmetric  shift_vec=[0 1 2 -1]  value=[zeros(2^(DSPB_MB_SS_param.FS), 1)]  inPortNames=['d1'; 'a1'; 'w1'; 'd2'; 'a2'; 'w2']  outPortNames=['q1'; 'q2']  dspbaimage=dspba_prim.jpg  text=fprintf('dmem%s',AdvDSPBDMemDisplay(UseDontCare));  style=Optimised  visibilities=8 + 1024 + 2^17 + 2^18  UseDontCare=on  TwinWritePorts=on  version=20141001
  EdgeDetect : DspbAdvFftLibrary/Common/EdgeDetect
  FIFO1 : DSPBAPrim/FIFO  primtype=fifo  nInputs=3  nOutputs=4  omode=Inherit via internal rule  otype=sfix(16)  scale=2^-15  rndmethod=Unbiased  factor=1  satmethod=Symmetric  shift_vec=[0 1 2 -1]  value=[2^(DSPB_MB_SS_param.FS) 1 2^(DSPB_MB_SS_param.FS)]  inPortNames=['w'; 'd'; 'r'; 'f']  outPortNames=['v'; 'q'; 't'; 'f']  dspbaimage=dspba_prim.jpg  text=fprintf('fifo');  style=Optimised  visibilities=263168  version=20130808  user_sclr=off
  GPIn : DSPBAPrim/GPIn  primtype=gpin  nInputs=evalAionMaskParam(gcb,'value',1)  nOutputs=evalAionMaskParam(gcb,'value',1)  omode=Inherit via internal rule  otype=sfix(16)  scale=2^-15  rndmethod=Unbiased  factor=1  satmethod=Symmetric  shift_vec=[0 1 2 -1]  value=4  inPortNames=[' ' ' ' ' ' ' ' ' ' ' ' ' ' ' ' ' ' ' ' ' ' ' ' ' ' ' ' ' ' ' ' ' ' ' ' ' ' ' ' ' ' ' ' ' ' ' ' ' ' ' ' ' ' ' ' ' ' ' ' ' ' ' ' ' ' ' ' ' ']'  outPortNames=[' ' ' ' ' ' ' ' ' ' ' ' ' ' ' ' ' ' ' ' ' ' ' ' ' ' ' ' ' ' ' ' ' ' ' ' ' ' ' ' ' ' ' ' ' ' ' ' ' ' ' ' ' ' ' ' ' ' ' ' ' ' ' ' ' ' ' ' ' ']'  dspbaimage=dspba_prim.jpg  text=fprintf('GPIn');  style=Optimised  visibilities=1024  latencyCorrection=0  scheduleOrigin=on  version=20090407
  GPOut : DSPBAPrim/GPOut  primtype=gpout  nInputs=evalAionMaskParam(gcb,'value',1)  nOutputs=evalAionMaskParam(gcb,'value',1)  omode=Inherit via internal rule  otype=sfix(16)  scale=2^-15  rndmethod=Unbiased  factor=1  satmethod=Symmetric  shift_vec=[0 1 2 -1]  value=2  inPortNames=[' ' ' ' ' ' ' ' ' ' ' ' ' ' ' ' ' ' ' ' ' ' ' ' ' ' ' ' ' ' ' ' ' ' ' ' ' ' ' ' ' ' ' ' ' ' ' ' ' ' ' ' ' ' ' ' ' ' ' ' ' ' ' ' ' ' ' ' ' ']'  outPortNames=[' ' ' ' ' ' ' ' ' ' ' ' ' ' ' ' ' ' ' ' ' ' ' ' ' ' ' ' ' ' ' ' ' ' ' ' ' ' ' ' ' ' ' ' ' ' ' ' ' ' ' ' ' ' ' ' ' ' ' ' ' ' ' ' ' ' ' ' ' ']'  dspbaimage=dspba_prim.jpg  text=fprintf('GPOut');  style=Optimised  visibilities=1024  latencyCorrection=0  version=20090407
  Mult : DSPBAPrim/Mult  primtype=mult  nInputs=2  nOutputs=1  omode=Inherit via internal rule  otype=sfix(16)  scale=2^-15  rndmethod=Unbiased  factor=1  satmethod=Symmetric  shift_vec=[0 1 2 -1]  value=0  inPortNames=[' '; ' ';]  outPortNames=[' ']  dspbaimage=dspba_prim.jpg  text=fprintf('X');  style=Optimised  visibilities=8+2^18+2^19  floatPrecision=float32_m23  floatRounding=correct  advOptions=[]  version=20130115
  Mult1 : DSPBAPrim/Mult  primtype=mult  nInputs=2  nOutputs=1  omode=Inherit via internal rule  otype=sfix(16)  scale=2^-15  rndmethod=Unbiased  factor=1  satmethod=Symmetric  shift_vec=[0 1 2 -1]  value=0  inPortNames=[' '; ' ';]  outPortNames=[' ']  dspbaimage=dspba_prim.jpg  text=fprintf('X');  style=Optimised  visibilities=8+2^18+2^19  floatPrecision=float32_m23  floatRounding=correct  advOptions=[]  version=20130115
  Mux : DSPBAPrim/Mux  primtype=mux  nInputs=evalAionMaskParam(gcb,'value',1)+1  nOutputs=1  omode=Inherit via internal rule  otype=sfix(16)  scale=2^-15  rndmethod=Unbiased  factor=1  satmethod=Symmetric  shift_vec=[0 1 2 -1]  value=2  inPortNames=['s '; 'd0'; 'd1'; 'd2'; 'd3'; 'd4'; 'd5'; 'd6'; 'd7'; 'd8'; 'd9';]  outPortNames=[' ']  dspbaimage=dspba_prim.jpg  text=fprintf('%s', primtype);  style=Optimised  visibilities=1032  version=20131025
  Mux1 : DSPBAPrim/Mux  primtype=mux  nInputs=evalAionMaskParam(gcb,'value',1)+1  nOutputs=1  omode=Inherit via internal rule  otype=sfix(16)  scale=2^-15  rndmethod=Unbiased  factor=1  satmethod=Symmetric  shift_vec=[0 1 2 -1]  value=2  inPortNames=['s '; 'd0'; 'd1'; 'd2'; 'd3'; 'd4'; 'd5'; 'd6'; 'd7'; 'd8'; 'd9';]  outPortNames=[' ']  dspbaimage=dspba_prim.jpg  text=fprintf('%s', primtype);  style=Optimised  visibilities=1032  version=20131025
  PulseMultiplier : DspbAdvFftLibrary/Common/PulseMultiplier  N=DSPB_MB_SS_param.FS
  Real-Imag to Complex : RealImagToComplex
  SampleDelay : DSPBAPrim/SampleDelay  primtype=sampdelay  nInputs=1  nOutputs=1  omode=Inherit via internal rule  otype=sfix(16)  scale=2^-15  rndmethod=Unbiased  factor=1  satmethod=Symmetric  shift_vec=[0 1 2 -1]  value=1  inPortNames=[' '; ' ';]  outPortNames=[' ']  dspbaimage=dspba_prim.jpg  text=dpoly(1, eye(1,value+1), 'z')  style=Optimised  visibilities=8 + 1024 + 2^17 + 2^18  flexible=off  slackgroup=0  augmented=0  version=20090407  advOptions=[]
  SynthesisInfo : DSPBAPrim/SynthesisInfo  primtype=synthinfo  nInputs=0  nOutputs=0  omode=Inherit via internal rule  otype=sfix(16)  scale=2^-15  rndmethod=Truncate  factor=1  satmethod=Symmetric  shift_vec=[0 1 2 -1]  value=99  inPortNames=[' '; ' ';]  outPortNames=[' ']  dspbaimage=dspba_prim_ctrl.jpg  text=fprintf('Style=%s', style);  style=Scheduled  visibilities=2^17+2^18+2^19+2^20  constraintInUse=off  constraintRelation=>  constraintLimit=2  bitAccurate=on  version=20150220
  Terminator1 : Terminator
  Terminator2 : Terminator
  Terminator3 : Terminator
  Trig : DSPBAPrim/Trig  primtype=trigfunc  nInputs=1  nOutputs=1  omode=Inherit via internal rule  otype=sfix(16)  scale=2^-15  rndmethod=Unbiased  factor=1  satmethod=Symmetric  shift_vec=[0 1 2 -1]  value=round([0:255]/17)  inPortNames=[' '; ' ';]  outPortNames=[' ']  dspbaimage=dspba_prim_float.jpg  text=fprintf('sin(a)');  style=Optimised  visibilities=2^17+2^18  functionExpr=cos(a)  advOptions=[struct('rangeReduction',0)]  version=20140803
  Trig1 : DSPBAPrim/Trig  primtype=trigfunc  nInputs=1  nOutputs=1  omode=Inherit via internal rule  otype=sfix(16)  scale=2^-15  rndmethod=Unbiased  factor=1  satmethod=Symmetric  shift_vec=[0 1 2 -1]  value=round([0:255]/17)  inPortNames=[' '; ' ';]  outPortNames=[' ']  dspbaimage=dspba_prim_float.jpg  text=fprintf('sin(a)');  style=Optimised  visibilities=2^17+2^18  functionExpr=sin(a)  advOptions=[struct('rangeReduction',0)]  version=20140803
  addr_counter : Subsystem
  addr_counter1 : Subsystem
  normalize : DSPBAPrim/Const Mult  primtype=constmult  nInputs=1  nOutputs=1  omode=Inherit via internal rule  otype=sfix(16)  scale=2^-15  rndmethod=Unbiased  factor=1  satmethod=Symmetric  shift_vec=[0 1 2 -1]  value=1/2^(DSPB_MB_SS_param.FS)  inPortNames=[' '; ' ';]  outPortNames=[' ']  dspbaimage=dspba_prim.jpg  text=fprintf('cx');  style=Optimised  visibilities=8+2^10+2^17+2^18  floatRounding=correct  advOptions=[]  version=20140218
  swap : DSPBAPrim/Sub  primtype=sub  nInputs=2  nOutputs=1  omode=Inherit via internal rule  otype=ufix(DSPB_MB_SS_param.FS+1)  scale=2^-0  rndmethod=Unbiased  factor=1  satmethod=Symmetric  shift_vec=[0 1 2 -1]  value=0  inPortNames=['+'; '-';]  outPortNames=[' ']  dspbaimage=dspba_prim.jpg  text=fprintf('-');  style=Optimised  visibilities=8+2^17+2^18  floatRounding=correct  advOptions=[]  version=20130115
  Output_Valid : Outport
  Output : Outport  Port=2
  wires:
  Enhanced_Magnitude_Valid/1 -> GPIn/1
  Enhanced_Magnitude/1 -> GPIn/2
  Phase_Valid/1 -> GPIn/3
  Phase/1 -> GPIn/4
  GPIn/4 -> FIFO1/2
  GPIn/3 -> FIFO1/1
  Const/1 -> CmpEQ1/1, swap/1
  addr_counter/1(count) -> Mux/2, swap/2, CmpEQ/2
  normalize/1 -> DualMem/1, DualMem/4
  Const1/1 -> CmpEQ/1
  And/1 -> And1/2, EdgeDetect/1
  EdgeDetect/1 -> And1/1
  And1/1 -> PulseMultiplier/1
  PulseMultiplier/1 -> SampleDelay/1
  Mux/1 -> DualMem/5
  addr_counter1/1(count) -> Mux/3
  DualMem/1 -> Terminator1/1
  FIFO1/3 -> Terminator2/1
  GPOut/2 -> Output/1
  FIFO1/4 -> Terminator3/1
  FIFO1/1 -> And/2
  CmpEQ/1 -> And/1
  swap/1 -> Mux1/2, CmpEQ1/2
  FIFO1/2 -> Trig1/1, Trig/1
  Trig1/1 -> Mult/2
  Real-Imag to Complex/1 -> GPOut/2
  Trig/1 -> Mult1/2
  Mult/1 -> Real-Imag to Complex/2
  DualMem/2 -> Mult/1, Mult1/1
  CmpEQ1/1 -> Mux1/1
  Mux1/1 -> DualMem/2
  Const2/1 -> Mux1/3
  Mult1/1 -> Real-Imag to Complex/1
  SampleDelay/1 -> addr_counter1/1(en), FIFO1/3, GPOut/1, Mux/1
  GPIn/2 -> normalize/1
  GPIn/1 -> DualMem/3, DualMem/6, addr_counter/1(en)
  GPOut/1 -> Output_Valid/1

== system DSPB_MB_SS/dut/Feature_Extraction/A_Posteriori_SNR/counter ==
  en : Inport
  CmpEQ : DSPBAPrim/CmpEQ  primtype=cmpeq  nInputs=2  nOutputs=1  omode=boolean  otype=sfix(16)  scale=2^-15  rndmethod=Unbiased  factor=1  satmethod=Symmetric  shift_vec=[0 1 2 -1]  value=0  inPortNames=[' '; ' ';]  outPortNames=[' ']  dspbaimage=dspba_prim.jpg  text=fprintf('==');  style=Optimised  visibilities=0  advOptions=[]  version=20130117
  Const1 : DSPBAPrim/Const  primtype=const  nInputs=0  nOutputs=1  omode=Specify via dialog  otype=ufix(DSPB_MB_SS_param.FS+1)  scale=2^-0  rndmethod=Unbiased  factor=1  satmethod=Symmetric  shift_vec=[0 1 2 -1]  value=2^(DSPB_MB_SS_param.FS-1)+1  inPortNames=['+'; '+';]  outPortNames=[' ']  dspbaimage=dspba_prim.jpg  text=fprintf('%s', num2str(value));  style=Optimised  visibilities=8 + 1024  floatPrecision=float32_m23  version=20120820
  Const2 : DSPBAPrim/Const  primtype=const  nInputs=0  nOutputs=1  omode=Specify via dialog  otype=ufix(DSPB_MB_SS_param.FS + 1)  scale=2^-0  rndmethod=Unbiased  factor=1  satmethod=Symmetric  shift_vec=[0 1 2 -1]  value=2^(DSPB_MB_SS_param.FS-1)  inPortNames=['+'; '+';]  outPortNames=[' ']  dspbaimage=dspba_prim.jpg  text=fprintf('%s', num2str(value));  style=Optimised  visibilities=8 + 1024  floatPrecision=float32_m23  version=20120820
  Const3 : DSPBAPrim/Const  primtype=const  nInputs=0  nOutputs=1  omode=boolean  otype=ufix(10)  scale=2^-0  rndmethod=Unbiased  factor=1  satmethod=Symmetric  shift_vec=[0 1 2 -1]  value=1  inPortNames=['+'; '+';]  outPortNames=[' ']  dspbaimage=dspba_prim.jpg  text=fprintf('%s', num2str(value));  style=Optimised  visibilities=8 + 1024  floatPrecision=float32_m23  version=20120820
  Const4 : DSPBAPrim/Const  primtype=const  nInputs=0  nOutputs=1  omode=Inherit via internal rule  otype=ufix(10)  scale=2^-0  rndmethod=Unbiased  factor=1  satmethod=Symmetric  shift_vec=[0 1 2 -1]  value=0  inPortNames=['+'; '+';]  outPortNames=[' ']  dspbaimage=dspba_prim.jpg  text=fprintf('%s', num2str(value));  style=Optimised  visibilities=8 + 1024  floatPrecision=float32_m23  version=20120820
  LoadableCounter : DSPBAPrim/LoadableCounter  primtype=loadablecounter  nInputs=5  nOutputs=1  omode=Specify via dialog  otype=ufix(DSPB_MB_SS_param.FS+1)  scale=2^-0  rndmethod=Unbiased  factor=1  satmethod=Symmetric  shift_vec=[0 1 2 -1]  value=[0 2^(DSPB_MB_SS_param.FS-1)+1 1]  inPortNames=['en';'ld';'i ';'s ';'m ']  outPortNames=[' ']  dspbaimage=dspba_prim.jpg  text=fprintf('loadable\ncounter\n[%d %d %d]', value(1), value(2), value(3));  style=Optimised  visibilities=8 + 1024  version=20090407
  SampleDelay : DSPBAPrim/SampleDelay  primtype=sampdelay  nInputs=1  nOutputs=1  omode=Inherit via internal rule  otype=sfix(16)  scale=2^-15  rndmethod=Unbiased  factor=1  satmethod=Symmetric  shift_vec=[0 1 2 -1]  value=1  inPortNames=[' '; ' ';]  outPortNames=[' ']  dspbaimage=dspba_prim.jpg  text=dpoly(1, eye(1,value+1), 'z')  style=Optimised  visibilities=8 + 1024 + 2^17 + 2^18  flexible=off  slackgroup=0  augmented=0  version=20090407  advOptions=[]
  count : Outport
  wires:
  Const2/1 -> CmpEQ/2
  CmpEQ/1 -> SampleDelay/1
  Const4/1 -> LoadableCounter/3
  Const1/1 -> LoadableCounter/5
  SampleDelay/1 -> LoadableCounter/2
  Const3/1 -> LoadableCounter/4
  en/1 -> LoadableCounter/1
  LoadableCounter/1 -> CmpEQ/1, count/1

== system DSPB_MB_SS/dut/Feature_Extraction/A_Posteriori_SNR/frame_fuse ==
  input : Inport
  CmpEQ : DSPBAPrim/CmpEQ  primtype=cmpeq  nInputs=2  nOutputs=1  omode=boolean  otype=sfix(16)  scale=2^-15  rndmethod=Unbiased  factor=1  satmethod=Symmetric  shift_vec=[0 1 2 -1]  value=0  inPortNames=[' '; ' ';]  outPortNames=[' ']  dspbaimage=dspba_prim.jpg  text=fprintf('==');  style=Optimised  visibilities=0  advOptions=[]  version=20130117
  Const : DSPBAPrim/Const  primtype=const  nInputs=0  nOutputs=1  omode=Inherit via internal rule  otype=sfix(16)  scale=2^-15  rndmethod=Unbiased  factor=1  satmethod=Symmetric  shift_vec=[0 1 2 -1]  value=2^(DSPB_MB_SS_param.FS-1)+1  inPortNames=['+'; '+';]  outPortNames=[' ']  dspbaimage=dspba_prim.jpg  text=fprintf('%s', num2str(value));  style=Optimised  visibilities=8 + 1024  floatPrecision=float32_m23  version=20120820
  Const1 : DSPBAPrim/Const  primtype=const  nInputs=0  nOutputs=1  omode=boolean  otype=sfix(16)  scale=2^-15  rndmethod=Unbiased  factor=1  satmethod=Symmetric  shift_vec=[0 1 2 -1]  value=0  inPortNames=['+'; '+';]  outPortNames=[' ']  dspbaimage=dspba_prim.jpg  text=fprintf('%s', num2str(value));  style=Optimised  visibilities=8 + 1024  floatPrecision=float32_m23  version=20120820
  Counter : DSPBAPrim/Counter  primtype=counter  nInputs=1  nOutputs=1  omode=Inherit via internal rule  otype=ufix(16)  scale=2^-0  rndmethod=Unbiased  factor=1  satmethod=Symmetric  shift_vec=[0 1 2 -1]  value=[0 2^(DSPB_MB_SS_param.FS-1)+2 1]  inPortNames=[' '; ' ';]  outPortNames=[' ']  dspbaimage=dspba_prim.jpg  text=fprintf('counter\n[%d %d %d]', value(1), value(2), value(3));  style=Optimised  visibilities=8 + 1024  version=20090407
  Mux : DSPBAPrim/Mux  primtype=mux  nInputs=evalAionMaskParam(gcb,'value',1)+1  nOutputs=1  omode=Inherit via internal rule  otype=sfix(16)  scale=2^-15  rndmethod=Unbiased  factor=1  satmethod=Symmetric  shift_vec=[0 1 2 -1]  value=2  inPortNames=['s '; 'd0'; 'd1'; 'd2'; 'd3'; 'd4'; 'd5'; 'd6'; 'd7'; 'd8'; 'd9';]  outPortNames=[' ']  dspbaimage=dspba_prim.jpg  text=fprintf('%s', primtype);  style=Optimised  visibilities=1032  version=20131025
  SampleDelay2 : DSPBAPrim/SampleDelay  primtype=sampdelay  nInputs=1  nOutputs=1  omode=Inherit via internal rule  otype=sfix(16)  scale=2^-15  rndmethod=Unbiased  factor=1  satmethod=Symmetric  shift_vec=[0 1 2 -1]  value=1  inPortNames=[' '; ' ';]  outPortNames=[' ']  dspbaimage=dspba_prim.jpg  text=dpoly(1, eye(1,value+1), 'z')  style=Optimised  visibilities=8 + 1024 + 2^17 + 2^18  flexible=off  slackgroup=0  augmented=0  version=20090407  advOptions=[]
  output : Outport
  wires:
  input/1 -> Mux/2
  Counter/1 -> CmpEQ/1
  Const/1 -> CmpEQ/2
  Mux/1 -> Counter/1
  CmpEQ/1 -> output/1, SampleDelay2/1
  SampleDelay2/1 -> Mux/1
  Const1/1 -> Mux/3
